simulink model "walkingRobotRL3D"  (R2020b)
settings: Solver=ode23t  StartTime=0.0  StopTime=Tf  RelTol=1e-2  EnableMultiTasking=on
PreLoadFcn:
  | robotParametersRL
undefined symbols (not defined in the file): agent, ankleD_pitch_jointMAX, ankleD_pitch_jointMIN, ankleD_roll_jointMAX, ankleD_roll_jointMIN, ankleI_pitch_jointMAX, ankleI_pitch_jointMIN, ankleI_roll_jointMAX, ankleI_roll_jointMIN, getSampleTime, height_plane, hipD_pitch_jointMAX, hipD_pitch_jointMIN, hipD_roll_jointMAX, hipD_roll_jointMIN, hipI_pitch_jointMAX, hipI_pitch_jointMIN, hipI_roll_jointMAX, hipI_roll_jointMIN, init_angs_L, init_angs_R, init_height, joint_damping, joint_limit_damping, joint_limit_stiffness, joint_stiffness, kneeD_jointMAX, kneeD_jointMIN, kneeI_jointMAX, kneeI_jointMIN, lower_leg_I0, lower_leg_length, lower_leg_mass, lower_leg_x, lower_leg_y, muscle_nominal_length, p10_ankleD_roll, plane_x, plane_y, regulator_type, tau, Tf, torso_height, torso_length, torso_offset_x, torso_offset_z, torso_width, torso_x, torso_y, torso_z, Ts, upper_leg_I0, upper_leg_length, upper_leg_mass, upper_leg_x, upper_leg_y, v10_ankleD_pitch, v10_ankleD_roll, v10_ankleI_pitch, v10_ankleI_roll ... (+41)
libraries: sm_lib x222, simulink x183, nesl_utility x130, walkingRobotUtils x69, rllib x2
(part 7 of 24)

== system walkingRobotRL3D/Walking Robot2/Robot Leg L ==
  torques : Inport
  Ankle Pitch to Roll : sm_lib/Frames and Transforms/Rigid Transform  TranslationMethod=None  TranslationStandardOffset=0  TranslationLengthUnit=m  TranslationStandardAxis=+Z  TranslationCartesianOffset=[0 0 0]  TranslationROffset=0  TranslationROffsetUnits=m  TranslationZOffset=0  TranslationZOffsetUnits=m  TranslationThetaOffset=0  TranslationThetaOffsetUnits=deg  RotationMethod=StandardAxis  RotationAngleUnits=deg  RotationStandardAxis=+Y  RotationAngle=90  RotationArbitraryAxis=[0 0 1]  FollAlignAxisA=+X  BaseAlignAxisA=+Y  FollAlignAxisB=+Y  BaseAlignAxisB=+Z  RotationSequenceAxes=FollowerAxes  RotationSequence=XYX  RotationSequenceAngles=[0 0 0]  RotationSequenceAnglesUnits=deg  RotationMatrix=[1 0 0; 0 1 0; 0 0 1]
  Ankle Roll to Pitch : sm_lib/Frames and Transforms/Rigid Transform  TranslationMethod=None  TranslationStandardOffset=0  TranslationLengthUnit=m  TranslationStandardAxis=+Z  TranslationCartesianOffset=[0 0 0]  TranslationROffset=0  TranslationROffsetUnits=m  TranslationZOffset=0  TranslationZOffsetUnits=m  TranslationThetaOffset=0  TranslationThetaOffsetUnits=deg  RotationMethod=StandardAxis  RotationAngleUnits=deg  RotationStandardAxis=+Y  RotationAngle=-90  RotationArbitraryAxis=[0 0 1]  FollAlignAxisA=+X  BaseAlignAxisA=+Y  FollAlignAxisB=+Y  BaseAlignAxisB=+Z  RotationSequenceAxes=FollowerAxes  RotationSequence=XYX  RotationSequenceAngles=[0 0 0]  RotationSequenceAnglesUnits=deg  RotationMatrix=[1 0 0; 0 1 0; 0 0 1]
  Ankle Pitch Joint : walkingRobotUtils/Leg Joint with Limits  VariantControl=actuatorType == 2  k=joint_stiffness  d=joint_damping  initAngle=init_angs_L(2)  eqAngle=0  upperLimit=ankleI_pitch_jointMAX  lowerLimit=ankleI_pitch_jointMIN  jointLimitStiffness=joint_limit_stiffness  jointLimitDamping=joint_limit_damping
  Ankle Roll Joint : walkingRobotUtils/Leg Joint with Limits  VariantControl=actuatorType == 2  k=joint_stiffness  d=joint_damping  initAngle=init_angs_L(1)  eqAngle=0  upperLimit=ankleI_roll_jointMAX  lowerLimit=ankleI_roll_jointMIN  jointLimitStiffness=joint_limit_stiffness  jointLimitDamping=joint_limit_damping
  Ankle to Lower Leg : sm_lib/Frames and Transforms/Rigid Transform  TranslationMethod=Cartesian  TranslationStandardOffset=0  TranslationLengthUnit=m  TranslationStandardAxis=+Z  TranslationCartesianOffset=[0 lower_leg_length/2 0]  TranslationROffset=0  TranslationROffsetUnits=m  TranslationZOffset=0  TranslationZOffsetUnits=m  TranslationThetaOffset=0  TranslationThetaOffsetUnits=deg  RotationMethod=StandardAxis  RotationAngleUnits=deg  RotationStandardAxis=+X  RotationAngle=-90  RotationArbitraryAxis=[0 0 1]  FollAlignAxisA=+X  BaseAlignAxisA=+Y  FollAlignAxisB=+Y  BaseAlignAxisB=+Z  RotationSequenceAxes=FollowerAxes  RotationSequence=XYX  RotationSequenceAngles=[0 0 0]  RotationSequenceAnglesUnits=deg  RotationMatrix=[1 0 0; 0 1 0; 0 0 1]
  Demux : Demux  Outputs=5
  Foot Offset : sm_lib/Frames and Transforms/Rigid Transform  TranslationMethod=Cartesian  TranslationStandardOffset=0  TranslationLengthUnit=m  TranslationStandardAxis=+Z  TranslationCartesianOffset=foot_offset  TranslationROffset=0  TranslationROffsetUnits=m  TranslationZOffset=0  TranslationZOffsetUnits=m  TranslationThetaOffset=0  TranslationThetaOffsetUnits=deg  RotationMethod=None  RotationAngleUnits=deg  RotationStandardAxis=+X  RotationAngle=-90  RotationArbitraryAxis=[0 0 1]  FollAlignAxisA=+X  BaseAlignAxisA=+Y  FollAlignAxisB=+Y  BaseAlignAxisB=+Z  RotationSequenceAxes=FollowerAxes  RotationSequence=XYX  RotationSequenceAngles=[0 0 0]  RotationSequenceAnglesUnits=deg  RotationMatrix=[1 0 0; 0 1 0; 0 0 1]
  Foot and Contact : walkingRobotUtils/Walking Robot (Control Design)/Robot Leg R/Foot and Contact  SystemSampleTime=-1  VariantActivationTime=update diagram  Latency=0  AutoFrameSizeCalculation=off
      link override Foot: CenterOfMass=foot_com  InertiaType=Custom  Mass=foot_mass  GraphicDiffuseColor=[1.0 0.0 0.0]  MomentsOfInertia=[foot_I0 foot_I0 foot_I0]  BrickDimensionUnits=m
      link override Spherical Solid: SphereRadiusUnits=m
      link override Spherical Solid1: SphereRadiusUnits=m
      link override Spherical Solid2: SphereRadiusUnits=m
      link override Spherical Solid3: SphereRadiusUnits=m
  Hip Pitch to Roll : sm_lib/Frames and Transforms/Rigid Transform  TranslationMethod=None  TranslationStandardOffset=0  TranslationLengthUnit=m  TranslationStandardAxis=+Z  TranslationCartesianOffset=[0 0 0]  TranslationROffset=0  TranslationROffsetUnits=m  TranslationZOffset=0  TranslationZOffsetUnits=m  TranslationThetaOffset=0  TranslationThetaOffsetUnits=deg  RotationMethod=StandardAxis  RotationAngleUnits=deg  RotationStandardAxis=+Y  RotationAngle=90  RotationArbitraryAxis=[0 0 1]  FollAlignAxisA=+X  BaseAlignAxisA=+Y  FollAlignAxisB=+Y  BaseAlignAxisB=+Z  RotationSequenceAxes=FollowerAxes  RotationSequence=XYX  RotationSequenceAngles=[0 0 0]  RotationSequenceAnglesUnits=deg  RotationMatrix=[1 0 0; 0 1 0; 0 0 1]
  Hip Roll to Pitch : sm_lib/Frames and Transforms/Rigid Transform  TranslationMethod=None  TranslationStandardOffset=0  TranslationLengthUnit=m  TranslationStandardAxis=+Z  TranslationCartesianOffset=[0 0 0]  TranslationROffset=0  TranslationROffsetUnits=m  TranslationZOffset=0  TranslationZOffsetUnits=m  TranslationThetaOffset=0  TranslationThetaOffsetUnits=deg  RotationMethod=StandardAxis  RotationAngleUnits=deg  RotationStandardAxis=+Y  RotationAngle=-90  RotationArbitraryAxis=[0 0 1]  FollAlignAxisA=+X  BaseAlignAxisA=+Y  FollAlignAxisB=+Y  BaseAlignAxisB=+Z  RotationSequenceAxes=FollowerAxes  RotationSequence=XYX  RotationSequenceAngles=[0 0 0]  RotationSequenceAnglesUnits=deg  RotationMatrix=[1 0 0; 0 1 0; 0 0 1]
  Hip Pitch Joint : walkingRobotUtils/Leg Joint with Limits  VariantControl=actuatorType == 2  k=joint_stiffness  d=joint_damping  initAngle=init_angs_L(5)  eqAngle=0  upperLimit=hipI_pitch_jointMAX  lowerLimit=hipI_pitch_jointMIN  jointLimitStiffness=joint_limit_stiffness  jointLimitDamping=joint_limit_damping
  Hip Roll Joint : walkingRobotUtils/Leg Joint with Limits  VariantControl=actuatorType == 2  k=joint_stiffness  d=joint_damping  initAngle=init_angs_L(4)  eqAngle=0  upperLimit=hipI_roll_jointMAX  lowerLimit=hipI_roll_jointMIN  jointLimitStiffness=joint_limit_stiffness  jointLimitDamping=joint_limit_damping
  Hip to World Coords : sm_lib/Frames and Transforms/Rigid Transform  TranslationMethod=None  TranslationStandardOffset=0  TranslationLengthUnit=cm  TranslationStandardAxis=+Z  TranslationCartesianOffset=[0 0 upper_leg_length/2]  TranslationROffset=0  TranslationROffsetUnits=m  TranslationZOffset=0  TranslationZOffsetUnits=m  TranslationThetaOffset=0  TranslationThetaOffsetUnits=deg  RotationMethod=StandardAxis  RotationAngleUnits=deg  RotationStandardAxis=+X  RotationAngle=-90  RotationArbitraryAxis=[0 0 1]  FollAlignAxisA=+X  BaseAlignAxisA=+Y  FollAlignAxisB=+Y  BaseAlignAxisB=+Z  RotationSequenceAxes=FollowerAxes  RotationSequence=XYX  RotationSequenceAngles=[0 0 0]  RotationSequenceAnglesUnits=deg  RotationMatrix=[1 0 0; 0 1 0; 0 0 1]
  Knee Joint : walkingRobotUtils/Leg Joint with Limits  VariantControl=actuatorType == 2  k=joint_stiffness  d=joint_damping  initAngle=init_angs_L(3)  eqAngle=0  upperLimit=kneeI_jointMAX  lowerLimit=kneeI_jointMIN  jointLimitStiffness=joint_limit_stiffness  jointLimitDamping=joint_limit_damping
  Knee to Upper Leg : sm_lib/Frames and Transforms/Rigid Transform  TranslationMethod=Cartesian  TranslationStandardOffset=0  TranslationLengthUnit=m  TranslationStandardAxis=+Z  TranslationCartesianOffset=[0 upper_leg_length/2 0]  TranslationROffset=0  TranslationROffsetUnits=m  TranslationZOffset=0  TranslationZOffsetUnits=m  TranslationThetaOffset=0  TranslationThetaOffsetUnits=deg  RotationMethod=StandardAxis  RotationAngleUnits=deg  RotationStandardAxis=+X  RotationAngle=-90  RotationArbitraryAxis=[0 0 1]  FollAlignAxisA=+X  BaseAlignAxisA=+Y  FollAlignAxisB=+Y  BaseAlignAxisB=+Z  RotationSequenceAxes=FollowerAxes  RotationSequence=XYX  RotationSequenceAngles=[0 0 0]  RotationSequenceAnglesUnits=deg  RotationMatrix=[1 0 0; 0 1 0; 0 0 1]
  Lower Leg : sm_lib/Body Elements/Brick Solid  GraphicAmbientColor=[0.15 0.15 0.15 1.0]  BasedOnType=Density  BrickDimensions=[lower_leg_x lower_leg_y lower_leg_length]  BrickDimensionUnits=m  CenterOfMass=lower_leg_com  CenterOfMassUnits=m  GraphicDiffuseColor=[0.2 1.0 0.2]  Density=1000  DensityUnits=kg/m^3  DoExposeReferenceFrame=on  GraphicEmissiveColor=[0.0 0.0 0.0 1.0]  ExportEntireGeometry=off  SerializedFrames=<Frames/>  MarkerShape=Sphere  MarkerSize=10  GraphicType=FromGeometry  InertiaType=Custom  Mass=lower_leg_mass  MassUnits=kg  MomentsOfInertia=[lower_leg_I0 lower_leg_I0 lower_leg_I0]  MomentsOfInertiaUnits=kg*m^2  GraphicOpacity=1.0  ProductsOfInertia=[0 0 0]  ProductsOfInertiaUnits=kg*m^2  GraphicShininess=75  GraphicSpecularColor=[0.5 0.5 0.5 1.0]  GraphicVisPropType=SimpleVisualProperties
  Lower Leg to Knee : sm_lib/Frames and Transforms/Rigid Transform  TranslationMethod=Cartesian  TranslationStandardOffset=0  TranslationLengthUnit=m  TranslationStandardAxis=+Z  TranslationCartesianOffset=[0 0 lower_leg_length/2]  TranslationROffset=0  TranslationROffsetUnits=m  TranslationZOffset=0  TranslationZOffsetUnits=m  TranslationThetaOffset=0  TranslationThetaOffsetUnits=deg  RotationMethod=StandardAxis  RotationAngleUnits=deg  RotationStandardAxis=+X  RotationAngle=90  RotationArbitraryAxis=[0 0 1]  FollAlignAxisA=+X  BaseAlignAxisA=+Y  FollAlignAxisB=+Y  BaseAlignAxisB=+Z  RotationSequenceAxes=FollowerAxes  RotationSequence=XYX  RotationSequenceAngles=[0 0 0]  RotationSequenceAnglesUnits=deg  RotationMatrix=[1 0 0; 0 1 0; 0 0 1]
  Package Measurements 3D : walkingRobotUtils/Package Measurements 3D  SystemSampleTime=-1  Latency=0  AutoFrameSizeCalculation=off
  Upper Leg : sm_lib/Body Elements/Brick Solid  GraphicAmbientColor=[0.15 0.15 0.15 1.0]  BasedOnType=Density  BrickDimensions=[upper_leg_x upper_leg_y upper_leg_length]  BrickDimensionUnits=m  CenterOfMass=upper_leg_com  CenterOfMassUnits=m  GraphicDiffuseColor=[0.0 0.0 1.0]  Density=1000  DensityUnits=kg/m^3  DoExposeReferenceFrame=on  GraphicEmissiveColor=[0.0 0.0 0.0 1.0]  ExportEntireGeometry=off  SerializedFrames=<Frames/>  MarkerShape=Sphere  MarkerSize=10  GraphicType=FromGeometry  InertiaType=Custom  Mass=upper_leg_mass  MassUnits=kg  MomentsOfInertia=[upper_leg_I0 upper_leg_I0 upper_leg_I0]  MomentsOfInertiaUnits=kg*m^2  GraphicOpacity=1.0  ProductsOfInertia=[0 0 0]  ProductsOfInertiaUnits=kg*m^2  GraphicShininess=75  GraphicSpecularColor=[0.5 0.5 0.5 1.0]  GraphicVisPropType=SimpleVisualProperties
  Upper Leg to Hip : sm_lib/Frames and Transforms/Rigid Transform  TranslationMethod=Cartesian  TranslationStandardOffset=0  TranslationLengthUnit=m  TranslationStandardAxis=+Z  TranslationCartesianOffset=[0 0 upper_leg_length/2]  TranslationROffset=0  TranslationROffsetUnits=m  TranslationZOffset=0  TranslationZOffsetUnits=m  TranslationThetaOffset=0  TranslationThetaOffsetUnits=deg  RotationMethod=StandardAxis  RotationAngleUnits=deg  RotationStandardAxis=+X  RotationAngle=90  RotationArbitraryAxis=[0 0 1]  FollAlignAxisA=+X  BaseAlignAxisA=+Y  FollAlignAxisB=+Y  BaseAlignAxisB=+Z  RotationSequenceAxes=FollowerAxes  RotationSequence=XYX  RotationSequenceAngles=[0 0 0]  RotationSequenceAnglesUnits=deg  RotationMatrix=[1 0 0; 0 1 0; 0 0 1]
  G : PMIOPort  Side=Right
  H : PMIOPort  Port=2  Side=Right
  meas : Outport  VectorParamsAs1DForOutWhenUnconnected=off
  wires:
  Ankle Roll Joint/1 -> Package Measurements 3D/3
  Hip Roll Joint/1 -> Package Measurements 3D/6
  Demux/5 -> Hip Pitch Joint/1
  Demux/4 -> Hip Roll Joint/1
  Demux/3 -> Knee Joint/1
  Demux/2 -> Ankle Pitch Joint/1
  Demux/1 -> Ankle Roll Joint/1
  torques/1 -> Demux/1
  Ankle Pitch Joint/1 -> Package Measurements 3D/4
  Package Measurements 3D/1 -> meas/1
  Hip Pitch Joint/1 -> Package Measurements 3D/7
  Knee Joint/1 -> Package Measurements 3D/5
  Foot and Contact/2 -> Package Measurements 3D/2
  Foot and Contact/1 -> Package Measurements 3D/1
  connections:
  Hip Roll to Pitch/RConn1 -- Hip Pitch Joint/LConn1
  Upper Leg to Hip/RConn1 -- Hip Pitch to Roll/LConn1
  Ankle Pitch Joint/LConn1 -- Ankle Roll to Pitch/RConn1
  Foot Offset/RConn1 -- Ankle Pitch to Roll/LConn1
  Hip Roll Joint/RConn1 -- Hip Roll to Pitch/LConn1
  Hip Roll Joint/LConn1 -- Hip Pitch to Roll/RConn1
  Hip Pitch Joint/RConn1 -- Hip to World Coords/LConn1
  Ankle Pitch Joint/RConn1 -- Ankle to Lower Leg/LConn1
  Ankle Roll Joint/RConn1 -- Ankle Roll to Pitch/LConn1
  Ankle Roll Joint/LConn1 -- Ankle Pitch to Roll/RConn1
  Knee Joint/RConn1 -- Knee to Upper Leg/LConn1
  G/RConn1 -- Foot and Contact/LConn1
  Ankle to Lower Leg/RConn1 -- Lower Leg/RConn1 -- Lower Leg to Knee/LConn1
  Upper Leg to Hip/LConn1 -- Upper Leg/RConn1 -- Knee to Upper Leg/RConn1
  Knee Joint/LConn1 -- Lower Leg to Knee/RConn1
  H/RConn1 -- Hip to World Coords/RConn1
  Foot and Contact/RConn1 -- Foot Offset/LConn1

== system walkingRobotRL3D/Walking Robot2/Robot Leg L1 ==
  torques : Inport
  Ankle Pitch to Roll : sm_lib/Frames and Transforms/Rigid Transform  TranslationMethod=None  TranslationStandardOffset=0  TranslationLengthUnit=m  TranslationStandardAxis=+Z  TranslationCartesianOffset=[0 0 0]  TranslationROffset=0  TranslationROffsetUnits=m  TranslationZOffset=0  TranslationZOffsetUnits=m  TranslationThetaOffset=0  TranslationThetaOffsetUnits=deg  RotationMethod=StandardAxis  RotationAngleUnits=deg  RotationStandardAxis=+Y  RotationAngle=90  RotationArbitraryAxis=[0 0 1]  FollAlignAxisA=+X  BaseAlignAxisA=+Y  FollAlignAxisB=+Y  BaseAlignAxisB=+Z  RotationSequenceAxes=FollowerAxes  RotationSequence=XYX  RotationSequenceAngles=[0 0 0]  RotationSequenceAnglesUnits=deg  RotationMatrix=[1 0 0; 0 1 0; 0 0 1]
  Ankle Roll to Pitch : sm_lib/Frames and Transforms/Rigid Transform  TranslationMethod=None  TranslationStandardOffset=0  TranslationLengthUnit=m  TranslationStandardAxis=+Z  TranslationCartesianOffset=[0 0 0]  TranslationROffset=0  TranslationROffsetUnits=m  TranslationZOffset=0  TranslationZOffsetUnits=m  TranslationThetaOffset=0  TranslationThetaOffsetUnits=deg  RotationMethod=StandardAxis  RotationAngleUnits=deg  RotationStandardAxis=+Y  RotationAngle=-90  RotationArbitraryAxis=[0 0 1]  FollAlignAxisA=+X  BaseAlignAxisA=+Y  FollAlignAxisB=+Y  BaseAlignAxisB=+Z  RotationSequenceAxes=FollowerAxes  RotationSequence=XYX  RotationSequenceAngles=[0 0 0]  RotationSequenceAnglesUnits=deg  RotationMatrix=[1 0 0; 0 1 0; 0 0 1]
  Ankle Pitch Joint : Subsystem  VariantControl=actuatorType == 2  mask(Leg Joint with Limits){k=joint_stiffness, d=joint_damping, initAngle=init_angs_L(2), eqAngle=0, upperLimit=ankleI_pitch_jointMAX, lowerLimit=ankleI_pitch_jointMIN, jointLimitStiffness=joint_limit_stiffness, jointLimitDamping=joint_limit_damping}
      mask prompts: k "Joint Stiffness [N*m/rad]"; d "Joint Damping [N*m/(rad/s)]"; initAngle "Initial Angle [rad]"; eqAngle "Equilibrium Angle [rad]"; upperLimit "Upper Angle Limit [rad]"; lowerLimit "Lower Angle Limit [rad]"; jointLimitStiffness "Joint Limit Stiffness [N*m/rad]"; jointLimitDamping "Joint Limit Damping [N*m/(rad/s)]"
      mask help: Torque-actuated revolute joint with limits and instrumented measurements.
      mask DialogControl DynamicsTab Prompt: Dynamics
      mask DialogControl LimitsTab Prompt: Limits
  Ankle Roll Joint : Subsystem  VariantControl=actuatorType == 2  mask(Leg Joint with Limits){k=joint_stiffness, d=joint_damping, initAngle=init_angs_L(1), eqAngle=0, upperLimit=ankleI_roll_jointMAX, lowerLimit=ankleI_roll_jointMIN, jointLimitStiffness=joint_limit_stiffness, jointLimitDamping=joint_limit_damping}
      mask prompts: k "Joint Stiffness [N*m/rad]"; d "Joint Damping [N*m/(rad/s)]"; initAngle "Initial Angle [rad]"; eqAngle "Equilibrium Angle [rad]"; upperLimit "Upper Angle Limit [rad]"; lowerLimit "Lower Angle Limit [rad]"; jointLimitStiffness "Joint Limit Stiffness [N*m/rad]"; jointLimitDamping "Joint Limit Damping [N*m/(rad/s)]"
      mask help: Torque-actuated revolute joint with limits and instrumented measurements.
      mask DialogControl DynamicsTab Prompt: Dynamics
      mask DialogControl LimitsTab Prompt: Limits
  Ankle to Lower Leg : sm_lib/Frames and Transforms/Rigid Transform  TranslationMethod=Cartesian  TranslationStandardOffset=0  TranslationLengthUnit=m  TranslationStandardAxis=+Z  TranslationCartesianOffset=[0 lower_leg_length/2 0]  TranslationROffset=0  TranslationROffsetUnits=m  TranslationZOffset=0  TranslationZOffsetUnits=m  TranslationThetaOffset=0  TranslationThetaOffsetUnits=deg  RotationMethod=StandardAxis  RotationAngleUnits=deg  RotationStandardAxis=+X  RotationAngle=-90  RotationArbitraryAxis=[0 0 1]  FollAlignAxisA=+X  BaseAlignAxisA=+Y  FollAlignAxisB=+Y  BaseAlignAxisB=+Z  RotationSequenceAxes=FollowerAxes  RotationSequence=XYX  RotationSequenceAngles=[0 0 0]  RotationSequenceAnglesUnits=deg  RotationMatrix=[1 0 0; 0 1 0; 0 0 1]
  Demux : Demux  Outputs=5
  Foot Offset : sm_lib/Frames and Transforms/Rigid Transform  TranslationMethod=Cartesian  TranslationStandardOffset=0  TranslationLengthUnit=m  TranslationStandardAxis=+Z  TranslationCartesianOffset=foot_offset  TranslationROffset=0  TranslationROffsetUnits=m  TranslationZOffset=0  TranslationZOffsetUnits=m  TranslationThetaOffset=0  TranslationThetaOffsetUnits=deg  RotationMethod=None  RotationAngleUnits=deg  RotationStandardAxis=+X  RotationAngle=-90  RotationArbitraryAxis=[0 0 1]  FollAlignAxisA=+X  BaseAlignAxisA=+Y  FollAlignAxisB=+Y  BaseAlignAxisB=+Z  RotationSequenceAxes=FollowerAxes  RotationSequence=XYX  RotationSequenceAngles=[0 0 0]  RotationSequenceAnglesUnits=deg  RotationMatrix=[1 0 0; 0 1 0; 0 0 1]
  Foot and Contact : walkingRobotUtils/Walking Robot (Control Design)/Robot Leg R/Foot and Contact  SystemSampleTime=-1  Latency=0  AutoFrameSizeCalculation=off
      link override Foot: CenterOfMass=foot_com  InertiaType=Custom  Mass=foot_mass  GraphicDiffuseColor=[1.0 0.0 0.0]  MomentsOfInertia=[foot_I0 foot_I0 foot_I0]  BrickDimensionUnits=m
      link override Spherical Solid: SphereRadiusUnits=m
      link override Spherical Solid1: SphereRadiusUnits=m
      link override Spherical Solid2: SphereRadiusUnits=m
      link override Spherical Solid3: SphereRadiusUnits=m
  Hip Pitch to Roll : sm_lib/Frames and Transforms/Rigid Transform  TranslationMethod=None  TranslationStandardOffset=0  TranslationLengthUnit=m  TranslationStandardAxis=+Z  TranslationCartesianOffset=[0 0 0]  TranslationROffset=0  TranslationROffsetUnits=m  TranslationZOffset=0  TranslationZOffsetUnits=m  TranslationThetaOffset=0  TranslationThetaOffsetUnits=deg  RotationMethod=StandardAxis  RotationAngleUnits=deg  RotationStandardAxis=+Y  RotationAngle=90  RotationArbitraryAxis=[0 0 1]  FollAlignAxisA=+X  BaseAlignAxisA=+Y  FollAlignAxisB=+Y  BaseAlignAxisB=+Z  RotationSequenceAxes=FollowerAxes  RotationSequence=XYX  RotationSequenceAngles=[0 0 0]  RotationSequenceAnglesUnits=deg  RotationMatrix=[1 0 0; 0 1 0; 0 0 1]
  Hip Roll to Pitch : sm_lib/Frames and Transforms/Rigid Transform  TranslationMethod=None  TranslationStandardOffset=0  TranslationLengthUnit=m  TranslationStandardAxis=+Z  TranslationCartesianOffset=[0 0 0]  TranslationROffset=0  TranslationROffsetUnits=m  TranslationZOffset=0  TranslationZOffsetUnits=m  TranslationThetaOffset=0  TranslationThetaOffsetUnits=deg  RotationMethod=StandardAxis  RotationAngleUnits=deg  RotationStandardAxis=+Y  RotationAngle=-90  RotationArbitraryAxis=[0 0 1]  FollAlignAxisA=+X  BaseAlignAxisA=+Y  FollAlignAxisB=+Y  BaseAlignAxisB=+Z  RotationSequenceAxes=FollowerAxes  RotationSequence=XYX  RotationSequenceAngles=[0 0 0]  RotationSequenceAnglesUnits=deg  RotationMatrix=[1 0 0; 0 1 0; 0 0 1]
  Hip Pitch Joint : Subsystem  VariantControl=actuatorType == 2  mask(Leg Joint with Limits){k=joint_stiffness, d=joint_damping, initAngle=init_angs_L(5), eqAngle=0, upperLimit=hipI_pitch_jointMAX, lowerLimit=hipI_pitch_jointMIN, jointLimitStiffness=joint_limit_stiffness, jointLimitDamping=joint_limit_damping}
      mask prompts: k "Joint Stiffness [N*m/rad]"; d "Joint Damping [N*m/(rad/s)]"; initAngle "Initial Angle [rad]"; eqAngle "Equilibrium Angle [rad]"; upperLimit "Upper Angle Limit [rad]"; lowerLimit "Lower Angle Limit [rad]"; jointLimitStiffness "Joint Limit Stiffness [N*m/rad]"; jointLimitDamping "Joint Limit Damping [N*m/(rad/s)]"
      mask help: Torque-actuated revolute joint with limits and instrumented measurements.
      mask DialogControl DynamicsTab Prompt: Dynamics
      mask DialogControl LimitsTab Prompt: Limits
  Hip Roll Joint : Subsystem  VariantControl=actuatorType == 2  mask(Leg Joint with Limits){k=joint_stiffness, d=joint_damping, initAngle=init_angs_L(4), eqAngle=0, upperLimit=hipI_roll_jointMAX, lowerLimit=hipI_roll_jointMIN, jointLimitStiffness=joint_limit_stiffness, jointLimitDamping=joint_limit_damping}
      mask prompts: k "Joint Stiffness [N*m/rad]"; d "Joint Damping [N*m/(rad/s)]"; initAngle "Initial Angle [rad]"; eqAngle "Equilibrium Angle [rad]"; upperLimit "Upper Angle Limit [rad]"; lowerLimit "Lower Angle Limit [rad]"; jointLimitStiffness "Joint Limit Stiffness [N*m/rad]"; jointLimitDamping "Joint Limit Damping [N*m/(rad/s)]"
      mask help: Torque-actuated revolute joint with limits and instrumented measurements.
      mask DialogControl DynamicsTab Prompt: Dynamics
      mask DialogControl LimitsTab Prompt: Limits
  Hip to World Coords : sm_lib/Frames and Transforms/Rigid Transform  TranslationMethod=None  TranslationStandardOffset=0  TranslationLengthUnit=cm  TranslationStandardAxis=+Z  TranslationCartesianOffset=[0 0 upper_leg_length/2]  TranslationROffset=0  TranslationROffsetUnits=m  TranslationZOffset=0  TranslationZOffsetUnits=m  TranslationThetaOffset=0  TranslationThetaOffsetUnits=deg  RotationMethod=StandardAxis  RotationAngleUnits=deg  RotationStandardAxis=+X  RotationAngle=-90  RotationArbitraryAxis=[0 0 1]  FollAlignAxisA=+X  BaseAlignAxisA=+Y  FollAlignAxisB=+Y  BaseAlignAxisB=+Z  RotationSequenceAxes=FollowerAxes  RotationSequence=XYX  RotationSequenceAngles=[0 0 0]  RotationSequenceAnglesUnits=deg  RotationMatrix=[1 0 0; 0 1 0; 0 0 1]
  Knee Joint : Subsystem  VariantControl=actuatorType == 2  mask(Leg Joint with Limits){k=joint_stiffness, d=joint_damping, initAngle=init_angs_L(3), eqAngle=0, upperLimit=kneeI_jointMAX, lowerLimit=kneeI_jointMIN, jointLimitStiffness=joint_limit_stiffness, jointLimitDamping=joint_limit_damping}
      mask prompts: k "Joint Stiffness [N*m/rad]"; d "Joint Damping [N*m/(rad/s)]"; initAngle "Initial Angle [rad]"; eqAngle "Equilibrium Angle [rad]"; upperLimit "Upper Angle Limit [rad]"; lowerLimit "Lower Angle Limit [rad]"; jointLimitStiffness "Joint Limit Stiffness [N*m/rad]"; jointLimitDamping "Joint Limit Damping [N*m/(rad/s)]"
      mask help: Torque-actuated revolute joint with limits and instrumented measurements.
      mask DialogControl DynamicsTab Prompt: Dynamics
      mask DialogControl LimitsTab Prompt: Limits
  Knee to Upper Leg : sm_lib/Frames and Transforms/Rigid Transform  TranslationMethod=Cartesian  TranslationStandardOffset=0  TranslationLengthUnit=m  TranslationStandardAxis=+Z  TranslationCartesianOffset=[0 upper_leg_length/2 0]  TranslationROffset=0  TranslationROffsetUnits=m  TranslationZOffset=0  TranslationZOffsetUnits=m  TranslationThetaOffset=0  TranslationThetaOffsetUnits=deg  RotationMethod=StandardAxis  RotationAngleUnits=deg  RotationStandardAxis=+X  RotationAngle=-90  RotationArbitraryAxis=[0 0 1]  FollAlignAxisA=+X  BaseAlignAxisA=+Y  FollAlignAxisB=+Y  BaseAlignAxisB=+Z  RotationSequenceAxes=FollowerAxes  RotationSequence=XYX  RotationSequenceAngles=[0 0 0]  RotationSequenceAnglesUnits=deg  RotationMatrix=[1 0 0; 0 1 0; 0 0 1]
  Lower Leg : sm_lib/Body Elements/Brick Solid  GraphicAmbientColor=[0.15 0.15 0.15 1.0]  BasedOnType=Density  BrickDimensions=[lower_leg_x lower_leg_y lower_leg_length]  BrickDimensionUnits=m  CenterOfMass=lower_leg_com  CenterOfMassUnits=m  GraphicDiffuseColor=[0.2 1.0 0.2]  Density=1000  DensityUnits=kg/m^3  DoExposeReferenceFrame=on  GraphicEmissiveColor=[0.0 0.0 0.0 1.0]  ExportEntireGeometry=off  SerializedFrames=<Frames/>  MarkerShape=Sphere  MarkerSize=10  GraphicType=FromGeometry  InertiaType=Custom  Mass=lower_leg_mass  MassUnits=kg  MomentsOfInertia=[lower_leg_I0 lower_leg_I0 lower_leg_I0]  MomentsOfInertiaUnits=kg*m^2  GraphicOpacity=1.0  ProductsOfInertia=[0 0 0]  ProductsOfInertiaUnits=kg*m^2  GraphicShininess=75  GraphicSpecularColor=[0.5 0.5 0.5 1.0]  GraphicVisPropType=SimpleVisualProperties
  Lower Leg to Knee : sm_lib/Frames and Transforms/Rigid Transform  TranslationMethod=Cartesian  TranslationStandardOffset=0  TranslationLengthUnit=m  TranslationStandardAxis=+Z  TranslationCartesianOffset=[0 0 lower_leg_length/2]  TranslationROffset=0  TranslationROffsetUnits=m  TranslationZOffset=0  TranslationZOffsetUnits=m  TranslationThetaOffset=0  TranslationThetaOffsetUnits=deg  RotationMethod=StandardAxis  RotationAngleUnits=deg  RotationStandardAxis=+X  RotationAngle=90  RotationArbitraryAxis=[0 0 1]  FollAlignAxisA=+X  BaseAlignAxisA=+Y  FollAlignAxisB=+Y  BaseAlignAxisB=+Z  RotationSequenceAxes=FollowerAxes  RotationSequence=XYX  RotationSequenceAngles=[0 0 0]  RotationSequenceAnglesUnits=deg  RotationMatrix=[1 0 0; 0 1 0; 0 0 1]
  Package Measurements 3D : walkingRobotUtils/Package Measurements 3D  SystemSampleTime=-1  Latency=0  AutoFrameSizeCalculation=off
  Upper Leg : sm_lib/Body Elements/Brick Solid  GraphicAmbientColor=[0.15 0.15 0.15 1.0]  BasedOnType=Density  BrickDimensions=[upper_leg_x upper_leg_y upper_leg_length]  BrickDimensionUnits=m  CenterOfMass=upper_leg_com  CenterOfMassUnits=m  GraphicDiffuseColor=[0.0 0.0 1.0]  Density=1000  DensityUnits=kg/m^3  DoExposeReferenceFrame=on  GraphicEmissiveColor=[0.0 0.0 0.0 1.0]  ExportEntireGeometry=off  SerializedFrames=<Frames/>  MarkerShape=Sphere  MarkerSize=10  GraphicType=FromGeometry  InertiaType=Custom  Mass=upper_leg_mass  MassUnits=kg  MomentsOfInertia=[upper_leg_I0 upper_leg_I0 upper_leg_I0]  MomentsOfInertiaUnits=kg*m^2  GraphicOpacity=1.0  ProductsOfInertia=[0 0 0]  ProductsOfInertiaUnits=kg*m^2  GraphicShininess=75  GraphicSpecularColor=[0.5 0.5 0.5 1.0]  GraphicVisPropType=SimpleVisualProperties
  Upper Leg to Hip : sm_lib/Frames and Transforms/Rigid Transform  TranslationMethod=Cartesian  TranslationStandardOffset=0  TranslationLengthUnit=m  TranslationStandardAxis=+Z  TranslationCartesianOffset=[0 0 upper_leg_length/2]  TranslationROffset=0  TranslationROffsetUnits=m  TranslationZOffset=0  TranslationZOffsetUnits=m  TranslationThetaOffset=0  TranslationThetaOffsetUnits=deg  RotationMethod=StandardAxis  RotationAngleUnits=deg  RotationStandardAxis=+X  RotationAngle=90  RotationArbitraryAxis=[0 0 1]  FollAlignAxisA=+X  BaseAlignAxisA=+Y  FollAlignAxisB=+Y  BaseAlignAxisB=+Z  RotationSequenceAxes=FollowerAxes  RotationSequence=XYX  RotationSequenceAngles=[0 0 0]  RotationSequenceAnglesUnits=deg  RotationMatrix=[1 0 0; 0 1 0; 0 0 1]
  G : PMIOPort  Side=Right
  H : PMIOPort  Port=2  Side=Right
  meas : Outport  VectorParamsAs1DForOutWhenUnconnected=off
  wires:
  Ankle Roll Joint/1(meas) -> Package Measurements 3D/3
  Hip Roll Joint/1(meas) -> Package Measurements 3D/6
  Demux/5 -> Hip Pitch Joint/1(t)
  Demux/4 -> Hip Roll Joint/1(t)
  Demux/3 -> Knee Joint/1(t)
  Demux/2 -> Ankle Pitch Joint/1(t)
  Demux/1 -> Ankle Roll Joint/1(t)
  torques/1 -> Demux/1
  Ankle Pitch Joint/1(meas) -> Package Measurements 3D/4
  Package Measurements 3D/1 -> meas/1
  Hip Pitch Joint/1(meas) -> Package Measurements 3D/7
  Knee Joint/1(meas) -> Package Measurements 3D/5
  Foot and Contact/2 -> Package Measurements 3D/2
  Foot and Contact/1 -> Package Measurements 3D/1
  connections:
  Hip Roll to Pitch/RConn1 -- Hip Pitch Joint/LConn1
  Upper Leg to Hip/RConn1 -- Hip Pitch to Roll/LConn1
  Ankle Pitch Joint/LConn1 -- Ankle Roll to Pitch/RConn1
  Foot Offset/RConn1 -- Ankle Pitch to Roll/LConn1
  Hip Roll Joint/RConn1 -- Hip Roll to Pitch/LConn1
  Hip Roll Joint/LConn1 -- Hip Pitch to Roll/RConn1
  Hip Pitch Joint/RConn1 -- Hip to World Coords/LConn1
  Ankle Pitch Joint/RConn1 -- Ankle to Lower Leg/LConn1
  Ankle Roll Joint/RConn1 -- Ankle Roll to Pitch/LConn1
  Ankle Roll Joint/LConn1 -- Ankle Pitch to Roll/RConn1
  Knee Joint/RConn1 -- Knee to Upper Leg/LConn1
  G/RConn1 -- Foot and Contact/LConn1
  Ankle to Lower Leg/RConn1 -- Lower Leg/RConn1 -- Lower Leg to Knee/LConn1
  Upper Leg to Hip/LConn1 -- Upper Leg/RConn1 -- Knee to Upper Leg/RConn1
  Knee Joint/LConn1 -- Lower Leg to Knee/RConn1
  H/RConn1 -- Hip to World Coords/RConn1
  Foot and Contact/RConn1 -- Foot Offset/LConn1

== system walkingRobotRL3D/Walking Robot2/Robot Leg R ==
  torques : Inport
  Ankle Pitch to Roll : sm_lib/Frames and Transforms/Rigid Transform  TranslationMethod=None  TranslationStandardOffset=0  TranslationLengthUnit=m  TranslationStandardAxis=+Z  TranslationCartesianOffset=[0 0 0]  TranslationROffset=0  TranslationROffsetUnits=m  TranslationZOffset=0  TranslationZOffsetUnits=m  TranslationThetaOffset=0  TranslationThetaOffsetUnits=deg  RotationMethod=StandardAxis  RotationAngleUnits=deg  RotationStandardAxis=+Y  RotationAngle=90  RotationArbitraryAxis=[0 0 1]  FollAlignAxisA=+X  BaseAlignAxisA=+Y  FollAlignAxisB=+Y  BaseAlignAxisB=+Z  RotationSequenceAxes=FollowerAxes  RotationSequence=XYX  RotationSequenceAngles=[0 0 0]  RotationSequenceAnglesUnits=deg  RotationMatrix=[1 0 0; 0 1 0; 0 0 1]
  Ankle Roll to Pitch : sm_lib/Frames and Transforms/Rigid Transform  TranslationMethod=None  TranslationStandardOffset=0  TranslationLengthUnit=m  TranslationStandardAxis=+Z  TranslationCartesianOffset=[0 0 0]  TranslationROffset=0  TranslationROffsetUnits=m  TranslationZOffset=0  TranslationZOffsetUnits=m  TranslationThetaOffset=0  TranslationThetaOffsetUnits=deg  RotationMethod=StandardAxis  RotationAngleUnits=deg  RotationStandardAxis=+Y  RotationAngle=-90  RotationArbitraryAxis=[0 0 1]  FollAlignAxisA=+X  BaseAlignAxisA=+Y  FollAlignAxisB=+Y  BaseAlignAxisB=+Z  RotationSequenceAxes=FollowerAxes  RotationSequence=XYX  RotationSequenceAngles=[0 0 0]  RotationSequenceAnglesUnits=deg  RotationMatrix=[1 0 0; 0 1 0; 0 0 1]
  Ankle Pitch Joint : walkingRobotUtils/Leg Joint with Limits  VariantControl=actuatorType == 2  k=joint_stiffness  d=joint_damping  initAngle=init_angs_R(2)  eqAngle=0  upperLimit=ankleD_pitch_jointMAX  lowerLimit=ankleD_pitch_jointMIN  jointLimitStiffness=joint_limit_stiffness  jointLimitDamping=joint_limit_damping
  Ankle Roll Joint : walkingRobotUtils/Leg Joint with Limits  VariantControl=actuatorType == 2  k=joint_stiffness  d=joint_damping  initAngle=init_angs_R(1)  eqAngle=0  upperLimit=ankleD_roll_jointMAX  lowerLimit=ankleD_roll_jointMIN  jointLimitStiffness=joint_limit_stiffness  jointLimitDamping=joint_limit_damping
  Ankle to Lower Leg : sm_lib/Frames and Transforms/Rigid Transform  TranslationMethod=Cartesian  TranslationStandardOffset=0  TranslationLengthUnit=m  TranslationStandardAxis=+Z  TranslationCartesianOffset=[0 lower_leg_length/2 0]  TranslationROffset=0  TranslationROffsetUnits=m  TranslationZOffset=0  TranslationZOffsetUnits=m  TranslationThetaOffset=0  TranslationThetaOffsetUnits=deg  RotationMethod=StandardAxis  RotationAngleUnits=deg  RotationStandardAxis=+X  RotationAngle=-90  RotationArbitraryAxis=[0 0 1]  FollAlignAxisA=+X  BaseAlignAxisA=+Y  FollAlignAxisB=+Y  BaseAlignAxisB=+Z  RotationSequenceAxes=FollowerAxes  RotationSequence=XYX  RotationSequenceAngles=[0 0 0]  RotationSequenceAnglesUnits=deg  RotationMatrix=[1 0 0; 0 1 0; 0 0 1]
  Demux : Demux  Outputs=5
  Foot Offset : sm_lib/Frames and Transforms/Rigid Transform  TranslationMethod=Cartesian  TranslationStandardOffset=0  TranslationLengthUnit=m  TranslationStandardAxis=+Z  TranslationCartesianOffset=foot_offset  TranslationROffset=0  TranslationROffsetUnits=m  TranslationZOffset=0  TranslationZOffsetUnits=m  TranslationThetaOffset=0  TranslationThetaOffsetUnits=deg  RotationMethod=None  RotationAngleUnits=deg  RotationStandardAxis=+X  RotationAngle=-90  RotationArbitraryAxis=[0 0 1]  FollAlignAxisA=+X  BaseAlignAxisA=+Y  FollAlignAxisB=+Y  BaseAlignAxisB=+Z  RotationSequenceAxes=FollowerAxes  RotationSequence=XYX  RotationSequenceAngles=[0 0 0]  RotationSequenceAnglesUnits=deg  RotationMatrix=[1 0 0; 0 1 0; 0 0 1]
  Foot and Contact : walkingRobotUtils/Walking Robot (Control Design)/Robot Leg R/Foot and Contact  SystemSampleTime=-1  VariantActivationTime=update diagram  Latency=0  AutoFrameSizeCalculation=off
      link override Foot: CenterOfMass=foot_com  GraphicDiffuseColor=[1.0 0.0 0.0]  InertiaType=Custom  Mass=foot_mass  MomentsOfInertia=[foot_I0 foot_I0 foot_I0]  BrickDimensionUnits=m
      link override Spherical Solid: SphereRadiusUnits=m
      link override Spherical Solid1: SphereRadiusUnits=m
      link override Spherical Solid2: SphereRadiusUnits=m
      link override Spherical Solid3: SphereRadiusUnits=m
  Hip Pitch to Roll : sm_lib/Frames and Transforms/Rigid Transform  TranslationMethod=None  TranslationStandardOffset=0  TranslationLengthUnit=m  TranslationStandardAxis=+Z  TranslationCartesianOffset=[0 0 0]  TranslationROffset=0  TranslationROffsetUnits=m  TranslationZOffset=0  TranslationZOffsetUnits=m  TranslationThetaOffset=0  TranslationThetaOffsetUnits=deg  RotationMethod=StandardAxis  RotationAngleUnits=deg  RotationStandardAxis=+Y  RotationAngle=90  RotationArbitraryAxis=[0 0 1]  FollAlignAxisA=+X  BaseAlignAxisA=+Y  FollAlignAxisB=+Y  BaseAlignAxisB=+Z  RotationSequenceAxes=FollowerAxes  RotationSequence=XYX  RotationSequenceAngles=[0 0 0]  RotationSequenceAnglesUnits=deg  RotationMatrix=[1 0 0; 0 1 0; 0 0 1]
  Hip Roll to Pitch : sm_lib/Frames and Transforms/Rigid Transform  TranslationMethod=None  TranslationStandardOffset=0  TranslationLengthUnit=m  TranslationStandardAxis=+Z  TranslationCartesianOffset=[0 0 0]  TranslationROffset=0  TranslationROffsetUnits=m  TranslationZOffset=0  TranslationZOffsetUnits=m  TranslationThetaOffset=0  TranslationThetaOffsetUnits=deg  RotationMethod=StandardAxis  RotationAngleUnits=deg  RotationStandardAxis=+Y  RotationAngle=-90  RotationArbitraryAxis=[0 0 1]  FollAlignAxisA=+X  BaseAlignAxisA=+Y  FollAlignAxisB=+Y  BaseAlignAxisB=+Z  RotationSequenceAxes=FollowerAxes  RotationSequence=XYX  RotationSequenceAngles=[0 0 0]  RotationSequenceAnglesUnits=deg  RotationMatrix=[1 0 0; 0 1 0; 0 0 1]
  Hip Pitch Joint : walkingRobotUtils/Leg Joint with Limits  VariantControl=actuatorType == 2  k=joint_stiffness  d=joint_damping  initAngle=init_angs_R(5)  eqAngle=0  upperLimit=hipD_pitch_jointMAX  lowerLimit=hipD_pitch_jointMIN  jointLimitStiffness=joint_limit_stiffness  jointLimitDamping=joint_limit_damping
  Hip Roll Joint : walkingRobotUtils/Leg Joint with Limits  VariantControl=actuatorType == 2  k=joint_stiffness  d=joint_damping  initAngle=init_angs_R(4)  eqAngle=0  upperLimit=hipD_roll_jointMAX  lowerLimit=hipD_roll_jointMIN  jointLimitStiffness=joint_limit_stiffness  jointLimitDamping=joint_limit_damping
  Hip to World Coords : sm_lib/Frames and Transforms/Rigid Transform  TranslationMethod=None  TranslationStandardOffset=0  TranslationLengthUnit=cm  TranslationStandardAxis=+Z  TranslationCartesianOffset=[0 0 upper_leg_length/2]  TranslationROffset=0  TranslationROffsetUnits=m  TranslationZOffset=0  TranslationZOffsetUnits=m  TranslationThetaOffset=0  TranslationThetaOffsetUnits=deg  RotationMethod=StandardAxis  RotationAngleUnits=deg  RotationStandardAxis=+X  RotationAngle=-90  RotationArbitraryAxis=[0 0 1]  FollAlignAxisA=+X  BaseAlignAxisA=+Y  FollAlignAxisB=+Y  BaseAlignAxisB=+Z  RotationSequenceAxes=FollowerAxes  RotationSequence=XYX  RotationSequenceAngles=[0 0 0]  RotationSequenceAnglesUnits=deg  RotationMatrix=[1 0 0; 0 1 0; 0 0 1]
  Knee Joint : walkingRobotUtils/Leg Joint with Limits  VariantControl=actuatorType == 2  k=joint_stiffness  d=joint_damping  initAngle=init_angs_R(3)  eqAngle=0  upperLimit=kneeD_jointMAX  lowerLimit=kneeD_jointMIN  jointLimitStiffness=joint_limit_stiffness  jointLimitDamping=joint_limit_damping
  Knee to Upper Leg : sm_lib/Frames and Transforms/Rigid Transform  TranslationMethod=Cartesian  TranslationStandardOffset=0  TranslationLengthUnit=m  TranslationStandardAxis=+Z  TranslationCartesianOffset=[0 upper_leg_length/2 0]  TranslationROffset=0  TranslationROffsetUnits=m  TranslationZOffset=0  TranslationZOffsetUnits=m  TranslationThetaOffset=0  TranslationThetaOffsetUnits=deg  RotationMethod=StandardAxis  RotationAngleUnits=deg  RotationStandardAxis=+X  RotationAngle=-90  RotationArbitraryAxis=[0 0 1]  FollAlignAxisA=+X  BaseAlignAxisA=+Y  FollAlignAxisB=+Y  BaseAlignAxisB=+Z  RotationSequenceAxes=FollowerAxes  RotationSequence=XYX  RotationSequenceAngles=[0 0 0]  RotationSequenceAnglesUnits=deg  RotationMatrix=[1 0 0; 0 1 0; 0 0 1]
  Lower Leg : sm_lib/Body Elements/Brick Solid  GraphicAmbientColor=[0.15 0.15 0.15 1.0]  BasedOnType=Density  BrickDimensions=[lower_leg_x lower_leg_y lower_leg_length]  BrickDimensionUnits=m  CenterOfMass=lower_leg_com  CenterOfMassUnits=m  GraphicDiffuseColor=[0.2 1.0 0.2]  Density=1000  DensityUnits=kg/m^3  DoExposeReferenceFrame=on  GraphicEmissiveColor=[0.0 0.0 0.0 1.0]  ExportEntireGeometry=off  SerializedFrames=<Frames/>  MarkerShape=Sphere  MarkerSize=10  GraphicType=FromGeometry  InertiaType=Custom  Mass=lower_leg_mass  MassUnits=kg  MomentsOfInertia=[lower_leg_I0 lower_leg_I0 lower_leg_I0]  MomentsOfInertiaUnits=kg*m^2  GraphicOpacity=1.0  ProductsOfInertia=[0 0 0]  ProductsOfInertiaUnits=kg*m^2  GraphicShininess=75  GraphicSpecularColor=[0.5 0.5 0.5 1.0]  GraphicVisPropType=SimpleVisualProperties
  Lower Leg to Knee : sm_lib/Frames and Transforms/Rigid Transform  TranslationMethod=Cartesian  TranslationStandardOffset=0  TranslationLengthUnit=m  TranslationStandardAxis=+Z  TranslationCartesianOffset=[0 0 lower_leg_length/2]  TranslationROffset=0  TranslationROffsetUnits=m  TranslationZOffset=0  TranslationZOffsetUnits=m  TranslationThetaOffset=0  TranslationThetaOffsetUnits=deg  RotationMethod=StandardAxis  RotationAngleUnits=deg  RotationStandardAxis=+X  RotationAngle=90  RotationArbitraryAxis=[0 0 1]  FollAlignAxisA=+X  BaseAlignAxisA=+Y  FollAlignAxisB=+Y  BaseAlignAxisB=+Z  RotationSequenceAxes=FollowerAxes  RotationSequence=XYX  RotationSequenceAngles=[0 0 0]  RotationSequenceAnglesUnits=deg  RotationMatrix=[1 0 0; 0 1 0; 0 0 1]
  Package Measurements 3D : walkingRobotUtils/Package Measurements 3D  SystemSampleTime=-1  Latency=0  AutoFrameSizeCalculation=off
  Upper Leg : sm_lib/Body Elements/Brick Solid  GraphicAmbientColor=[0.15 0.15 0.15 1.0]  BasedOnType=Density  BrickDimensions=[upper_leg_x upper_leg_y upper_leg_length]  BrickDimensionUnits=m  CenterOfMass=upper_leg_com  CenterOfMassUnits=m  GraphicDiffuseColor=[0.0 0.0 1.0]  Density=1000  DensityUnits=kg/m^3  DoExposeReferenceFrame=on  GraphicEmissiveColor=[0.0 0.0 0.0 1.0]  ExportEntireGeometry=off  SerializedFrames=<Frames/>  MarkerShape=Sphere  MarkerSize=10  GraphicType=FromGeometry  InertiaType=Custom  Mass=upper_leg_mass  MassUnits=kg  MomentsOfInertia=[upper_leg_I0 upper_leg_I0 upper_leg_I0]  MomentsOfInertiaUnits=kg*m^2  GraphicOpacity=1.0  ProductsOfInertia=[0 0 0]  ProductsOfInertiaUnits=kg*m^2  GraphicShininess=75  GraphicSpecularColor=[0.5 0.5 0.5 1.0]  GraphicVisPropType=SimpleVisualProperties
  Upper Leg to Hip : sm_lib/Frames and Transforms/Rigid Transform  TranslationMethod=Cartesian  TranslationStandardOffset=0  TranslationLengthUnit=m  TranslationStandardAxis=+Z  TranslationCartesianOffset=[0 0 upper_leg_length/2]  TranslationROffset=0  TranslationROffsetUnits=m  TranslationZOffset=0  TranslationZOffsetUnits=m  TranslationThetaOffset=0  TranslationThetaOffsetUnits=deg  RotationMethod=StandardAxis  RotationAngleUnits=deg  RotationStandardAxis=+X  RotationAngle=90  RotationArbitraryAxis=[0 0 1]  FollAlignAxisA=+X  BaseAlignAxisA=+Y  FollAlignAxisB=+Y  BaseAlignAxisB=+Z  RotationSequenceAxes=FollowerAxes  RotationSequence=XYX  RotationSequenceAngles=[0 0 0]  RotationSequenceAnglesUnits=deg  RotationMatrix=[1 0 0; 0 1 0; 0 0 1]
  G : PMIOPort  Side=Right
  H : PMIOPort  Port=2  Side=Right
  meas : Outport  VectorParamsAs1DForOutWhenUnconnected=off
  wires:
  Knee Joint/1 -> Package Measurements 3D/5
  Hip Pitch Joint/1 -> Package Measurements 3D/7
  Package Measurements 3D/1 -> meas/1
  Ankle Pitch Joint/1 -> Package Measurements 3D/4
  torques/1 -> Demux/1
  Demux/1 -> Ankle Roll Joint/1
  Demux/2 -> Ankle Pitch Joint/1
  Demux/3 -> Knee Joint/1
  Demux/4 -> Hip Roll Joint/1
  Demux/5 -> Hip Pitch Joint/1
  Hip Roll Joint/1 -> Package Measurements 3D/6
  Ankle Roll Joint/1 -> Package Measurements 3D/3
  Foot and Contact/2 -> Package Measurements 3D/2
  Foot and Contact/1 -> Package Measurements 3D/1
  connections:
  H/RConn1 -- Hip to World Coords/RConn1
  Knee Joint/LConn1 -- Lower Leg to Knee/RConn1
  Knee to Upper Leg/RConn1 -- Upper Leg/RConn1 -- Upper Leg to Hip/LConn1
  Lower Leg to Knee/LConn1 -- Lower Leg/RConn1 -- Ankle to Lower Leg/RConn1
  Knee Joint/RConn1 -- Knee to Upper Leg/LConn1
  Ankle Roll Joint/LConn1 -- Ankle Pitch to Roll/RConn1
  Ankle Roll Joint/RConn1 -- Ankle Roll to Pitch/LConn1
  Ankle Pitch Joint/RConn1 -- Ankle to Lower Leg/LConn1
  Hip Pitch Joint/RConn1 -- Hip to World Coords/LConn1
  Hip Roll Joint/LConn1 -- Hip Pitch to Roll/RConn1
  Hip Roll Joint/RConn1 -- Hip Roll to Pitch/LConn1
  Foot Offset/RConn1 -- Ankle Pitch to Roll/LConn1
  Ankle Pitch Joint/LConn1 -- Ankle Roll to Pitch/RConn1
  Upper Leg to Hip/RConn1 -- Hip Pitch to Roll/LConn1
  Hip Roll to Pitch/RConn1 -- Hip Pitch Joint/LConn1
  Foot and Contact/RConn1 -- Foot Offset/LConn1
  G/RConn1 -- Foot and Contact/LConn1
